simulink model "example_compound"  (Simulink 8.1)
settings: Solver=ode45  StartTime=0.0  StopTime=10.0  RelTol=1e-3
undefined symbols (not defined in the file): find_system
libraries: powerlib x6, powerlib_models x1
settings Model: Creator=gshah  LastModifiedBy=Yooshaa
settings OptimizationCC: ExpressionDepthLimit=128  InitFltsAndDblsToZero=on
settings DebuggingCC: SaveWithParameterizedLinksMsg=none  SignalResolutionControl=TryResolveAllWithWarning  MultiTaskDSMMsg=warning  MultiTaskCondExecSysMsg=none  StrictBusMsg=Warning
settings RTWCC: IncludeERTFirstTime=on
settings GRTTargetCC: TargetFcnLib=ansi_tfl_tmw.mat

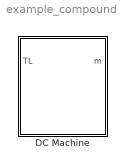
== system example_compound ==
  DC Machine : Subsystem  LoadFcn=find_system(gcs,'FollowLinks', 'on', 'LookUnderMasks', 'all');  mask(DC machine){PresetModel=No, MechanicalLoad=Torque TL, ShowDetailedParameters=on, RLa=[ 0.5  0.01], RLf=[ 240  120], Laf=1.8, J=0.05, Bm=0.02, Tf=0, w0=0}
      mask prompts: PresetModel "Preset  model"; MechanicalLoad "Mechanical input:"; ShowDetailedParameters "-----------------  Show detailed parameters -----------------"; RLa "Armature resistance and inductance [Ra (ohms) La (H) ]"; RLf "Field resistance and inductance [Rf (ohms) Lf (H) ]"; Laf "Field-armature mutual inductance Laf (H) :"; J "Total inertia J (kg.m^2)"; Bm "Viscous friction coefficient Bm (N.m.s)"; Tf "Coulomb friction torque Tf (N.m)"; w0 "Initial speed (rad/s) :"
      mask help: This block implements a separately excited DC machine. Access is provided to the field connections so that the machine can be used as a shunt-connected or a series-connected DC machine.
      mask init:
      | Ra=RLa(1); La=RLa(2);
      | Rf=RLf(1); Lf=RLf(2);
      | powericon('DCMachineInit',gcb,0);
      | power_initmask();
      settings: OpenFcn=power_openblockproxy();
      mask Help: web(psbhelp)
      mask TypeOptions PresetModel: No | 01: 5HP 240V 1750RPM Field:300V | 02: 5HP 240V 1750RPM Field:150V | 03: 5HP 500V 1750RPM Field:300V | 04: 10HP 240V 1750RPM Field:300V | 05: 10HP 500V 1750RPM Field:300V | 06: 20HP 240V 1750RPM Field:300V | 07: 20HP 500V 1750RPM Field:300V | 08: 30HP 240V 1750RPM Field:300V | 09: 30HP 500V 1750RPM Field:300V | 10: 40HP 240V 1750RPM Field:300V | 11: 40HP 500V 1750RPM Field:300V | 12: 50HP 240V 1750RPM Field:300V | 13: 50HP 500V 1750RPM Field:300V | 14: 75HP 500V 1750RPM Field:300V | 15: 100HP 500V 1750RPM Field:300V | 16: 125HP 500V 1750RPM Field:300V | 17: 150HP 500V 1750RPM Field:300V | 18: 175HP 500V 1750RPM Field:300V | 19: 200HP 440V 1184RPM Field:310V | 20: 200HP 500V 1750RPM Field:150V | 21: 200HP 500V 1750RPM Field:300V | 22: 225HP 500V 1750RPM Field:300V | 23: 250HP 500V 1750RPM Field:300V
      mask Callback PresetModel: powericon('DCMachineCback',gcb,'Continuous');
      mask TypeOptions MechanicalLoad: Torque TL | Speed w
      mask Callback MechanicalLoad: powericon('DCMachineCback',gcb,'Continuous');
      mask Callback ShowDetailedParameters: powericon('DCMachineCback',gcb,'Continuous');
      mask Display:
      | plot(-80,-80,80,80,[0,9,18,24,29,30,29,24,18,9,0,-9,-18,-24,-29,-30,-29,-24,-18,-9,0],[30,29,24,18,9,0,-9,-18,-24,-29,-30,-29,-24,-18,-9,0,9,18,24,29,30],[-29,-35,-35,-29],[-8,-8,8,8],[29,35,35,29],[-8,-8,8,8],[-35,-55],[0,0],[35,55],[0,0],[-78,-50,-50,-49,-45,-39,-33,-26,-21,-18,-17,-19,-22,-22,-26,-27,-25,-22,-16,-9,-3,2,6,6,4,1,1,-3,-4,-2,2,7,14,20,26,29,30,28,24,24,21,20,21,25,31,37,44,49,50,50,50,78]*.7,[58,58,57.2,49.2,42.8,38.8,38,39.6,44.4,51.6,59.6,67.6,72.4,72.4,65.2,57.2,49.2,42.8,38.8,38,39.6,44.4,51.6,59.6,67.6,72.4,72.4,65.2,57.2,49.2,42.8,38.8,38,39.6,44.4,51.6,59.6,67.6,72.4,72.4,65.2,57.2,49.2,42.8,38.8,38,39.6,44.4,51.6,58,58,58]*.6-85 );
      | 
      | disp('dc')
      | 
      | color('blue');
      | 
      | plot([-50,-10,-10],[50,50,30]);
      | 
      | plot([50,10,10],[50,50,30]);

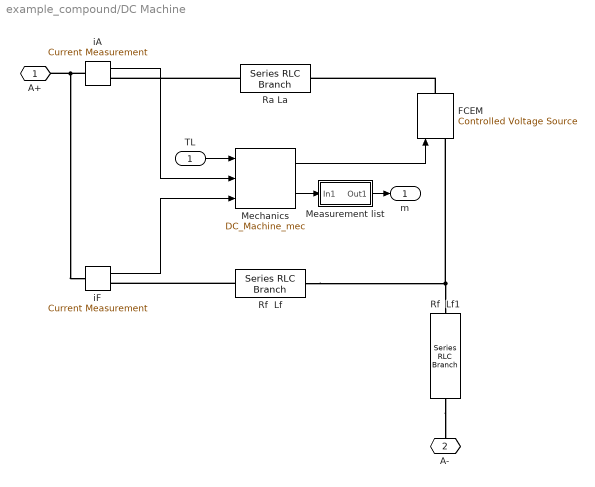
== system example_compound/DC Machine ==
  TL : Inport
  FCEM : powerlib/Electrical Sources/Controlled Voltage Source  Description=source block  Initialize=on  Source_Type=AC  Amplitude=0  Phase=0  Frequency=0  Measurements=None
  Measurement list : Subsystem
  Mechanics : powerlib_models/Continuous/DC_Machine_mec
  Ra La : powerlib/Elements/Series RLC Branch  LConnTagsString=__new0  RConnTagsString=__new0  BranchType=RL  Resistance=Ra  Inductance=La  SetiL0=off  InitialCurrent=0  Capacitance=inf  Setx0=off  InitialVoltage=0  Measurements=None
  Rf  Lf : powerlib/Elements/Series RLC Branch  LConnTagsString=__new0  RConnTagsString=__new0  BranchType=RL  Resistance=Rf  Inductance=Lf  SetiL0=off  InitialCurrent=0  Capacitance=inf  Setx0=off  InitialVoltage=0  Measurements=None
  Rf  Lf1 : powerlib/Elements/Series RLC Branch  LConnTagsString=__new0  RConnTagsString=__new0  BranchType=RL  Resistance=Rf  Inductance=Lf  SetiL0=off  InitialCurrent=0  Capacitance=inf  Setx0=off  InitialVoltage=0  Measurements=None
  iA : powerlib/Measurements/Current Measurement  PhasorSimulation=off  OutputType=Magnitude  PSBequivalent=0
  iF : powerlib/Measurements/Current Measurement  PhasorSimulation=off  OutputType=Magnitude  PSBequivalent=0
  A+ : PMIOPort  Port=1  Side=Left
  A- : PMIOPort  Port=2  Side=Right
  m : Outport
  wires:
  Measurement list/1(Out1) -> m/1
  iA/1 -> Mechanics/2
  Mechanics/1 -> FCEM/1
  iF/1 -> Mechanics/3
  TL/1 -> Mechanics/1
  Mechanics/2 -> Measurement list/1(In1)
  connections:
  iA/LConn1 -- A+/RConn1 -- iF/LConn1
  FCEM/RConn1 -- Ra La/RConn1
  Ra La/LConn1 -- iA/RConn1
  Rf  Lf/LConn1 -- iF/RConn1
  Rf  Lf/RConn1 -- FCEM/LConn1 -- Rf  Lf1/LConn1
  Rf  Lf1/RConn1 -- A-/RConn1

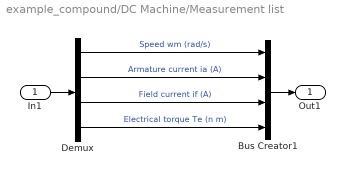
== system example_compound/DC Machine/Measurement list ==
  In1 : Inport
  Bus Creator1 : BusCreator
  Demux : Demux  Outputs=[1,1,1,1]
  Out1 : Outport
  wires:
  Demux/4 -> Bus Creator1/4  "Electrical torque Te (n m)"
  Demux/3 -> Bus Creator1/3  "Field current if (A)"
  Demux/2 -> Bus Creator1/2  "Armature current ia (A)"
  Demux/1 -> Bus Creator1/1  "Speed wm (rad/s)"
  Bus Creator1/1 -> Out1/1
  In1/1 -> Demux/1
